simulink model "untitled1"  (Simulink 6.0)
settings: Solver=ode45  StartTime=0.0  StopTime=2  RelTol=1e-3
libraries: powerlib x5, powerlib_extras x3, simulink x1
settings Model: Creator=Daniel  LastModifiedBy=GXP
settings OptimizationCC: InlineInvariantSignals=off  InitFltsAndDblsToZero=off
settings DebuggingCC: SignalResolutionControl=UseLocalSettings
settings GRTTargetCC: TargetFcnLib=ansi_tfl_table_tmw.mat

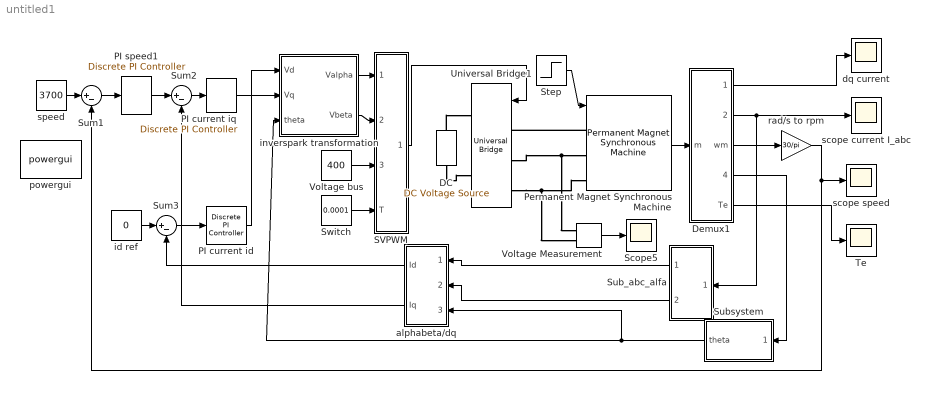
== system untitled1 ==
  " rad/s to rpm" : Gain  Gain=30/pi  ParameterDataType=fixdt(1, 16)  OutDataType=fixdt(1, 16)
  DC : powerlib/Electrical Sources/DC Voltage Source  Orientation=up  Amplitude=400  Measurements=Voltage
  Demux1 : Subsystem
  PI current id : powerlib_extras/Discrete  Control Blocks/Discrete PI Controller  Kp=100  Ki=7000  Par_Limits=[1000 -1000]  Init=0  Ts=50e-6
  PI current iq : powerlib_extras/Discrete  Control Blocks/Discrete PI Controller  Kp=100  Ki=7000  Par_Limits=[1000 -1000]  Init=0  Ts=50e-6
  PI speed1 : powerlib_extras/Discrete  Control Blocks/Discrete PI Controller  Kp=0.09  Ki=2.7  Par_Limits=[1500 -150]  Init=0  Ts=50e-6
  Permanent Magnet Synchronous Machine : powerlib/Machines/Permanent Magnet Synchronous Machine  PresetModel=No  ShowDetailedParameters=on  Resistance=1.08  Inductances=[8.5e-3, 8.5e-3]  Flux=0.1801  Mechanical=[0.00138 0.003 3]
  SVPWM : Subsystem
  Scope5 : Scope
      settings: TickLabels=on  TimeRange=2  YMin=-450  YMax=450  SaveName=ScopeData2  SampleInput=on
  Step : Step  Time=0.8  After=0  SampleTime=0
  Sub_abc_alfa : Subsystem  Orientation=left
  Subsystem : Subsystem  Orientation=left
  Sum1 : Sum  Inputs=|+-  OutDataType=fixdt(1, 16)
  Sum2 : Sum  Inputs=|+-  OutDataType=fixdt(1, 16)
  Sum3 : Sum  Inputs=|+-  OutDataType=fixdt(1, 16)
  Switch : Constant  Value=0.0001  VectorParams1D=off
  Te : Scope
      settings: TickLabels=on  TimeRange=1  YMin=1.9  YMax=2.5  SaveName=te3  SampleInput=on
  Universal Bridge1 : powerlib/Power Electronics/Universal Bridge  Orientation=left  Arms=3  SnubberResistance=1e5  SnubberCapacitance=inf  Device=IGBT / Diodes  Ron=1e-3  Lon=0  ForwardVoltages="[  0  0  ]"  ForwardVoltage=0  GTOparameters=[ 10e-6 , 20e-6 ]  IGBTparameters=[ 1e-6 , 2e-6 ]  Measurements=None
  Voltage Measurement : powerlib/Measurements/Voltage Measurement  PhasorSimulation=off  OutputType=Complex  PSBequivalent=0
  Voltage bus : Constant  Value=400  OutDataType=fixdt(1, 16)
  alphabeta/dq : Subsystem  Orientation=left
  dq current : Scope
      settings: TimeRange=2  YMin=-0.25  YMax=3.25  SaveName=ScopeData4  SampleInput=on
  id ref : Constant  Value=0
  inverspark transformation : Subsystem
  powergui : powerlib/powergui  Priority=2  Frange=[0:2:500]  Ylog=off  Xlog=on  save=off  variable=ZData  ZoomFFT=on  StartTime=0.0  cycles=1  DisplayStyle=1  fundamental=60  FreqAxis=off  MaxFrequency=1000  frequencyindice=0  frequencyindicesteady=1  RmsSteady=1  display=off  Ts=0  methode=off  frequency=60  echomessages=off
  scope current I_abc : Scope
      settings: TickLabels=on  TimeRange=2  YMin=-1.12119  YMax=0.92681  SaveName=ScopeData5  SampleInput=on
  scope speed : Scope
      settings: TimeRange=2  YMin=3740  YMax=3900  SaveName=ScopeData6  SampleInput=on
  speed : Constant  Value=3700
  wires:
  Sum1/1 -> PI speed1/1
  Sum2/1 -> PI current iq/1
  Sum3/1 -> PI current id/1
  Step/1 -> Permanent Magnet Synchronous Machine/1
  Voltage bus/1 -> SVPWM/3(Vdc)
  Switch/1 -> SVPWM/4(T)
  PI current id/1 -> inverspark transformation/1(Vd)
  PI current iq/1 -> inverspark transformation/2(Vq)
  Permanent Magnet Synchronous Machine/1 -> Demux1/1(m)
  Demux1/1(Is_dq) -> dq current/1
  Sub_abc_alfa/2(I_beeta) -> alphabeta/dq/2(I_beta)
  Demux1/4(theta) -> Subsystem/1(thetam)
  Demux1/2(Is_abc) -> Sub_abc_alfa/1(Is_abc), scope current I_abc/1
  Demux1/5(Te) -> Te/1
  Voltage Measurement/1 -> Scope5/1
  speed/1 -> Sum1/1
  Demux1/3(wm) -> " rad/s to rpm"/1
  " rad/s to rpm"/1 -> scope speed/1, Sum1/2
  inverspark transformation/1(Valpha) -> SVPWM/1(Valpha)
  inverspark transformation/2(Vbeta) -> SVPWM/2(Vbate)
  Subsystem/1(theta) -> alphabeta/dq/3(theta), inverspark transformation/3(theta)
  PI speed1/1 -> Sum2/1
  Sub_abc_alfa/1(I_alfa) -> alphabeta/dq/1(I_alpha)
  alphabeta/dq/1(Id) -> Sum3/2
  alphabeta/dq/2(Iq) -> Sum2/2
  SVPWM/1(Pules) -> Universal Bridge1/1
  id ref/1 -> Sum3/1
  connections:
  DC/RConn1 -- Universal Bridge1/RConn1
  DC/LConn1 -- Universal Bridge1/RConn2
  Universal Bridge1/LConn2 -- Permanent Magnet Synchronous Machine/LConn2 -- Voltage Measurement/LConn1
  Universal Bridge1/LConn3 -- Permanent Magnet Synchronous Machine/LConn3 -- Voltage Measurement/LConn2
  Permanent Magnet Synchronous Machine/LConn1 -- Universal Bridge1/LConn1

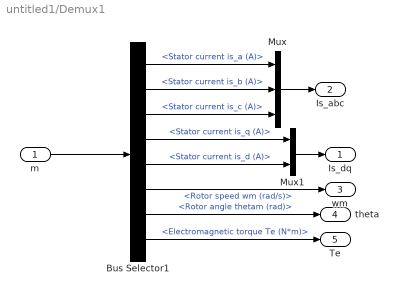
== system untitled1/Demux1 ==
  m : Inport  Port=1  LatchInput=off
  Bus Selector1 : BusSelector  DialogController=Simulink.DDGSource_Bus  OutputSignals=Stator current is_a (A),Stator current is_b (A),Stator current is_c (A),Stator current is_q (A),Stator current is_d (A),Rotor speed wm (rad/s),Rotor angle thetam (rad),Electromagnetic torque Te (N*m)
  Mux : Mux  Inputs=3
  Mux1 : Mux  Inputs=2
  Is_dq : Outport
  Is_abc : Outport  Port=2
  wm : Outport  Port=3
  theta : Outport  Port=4
  Te : Outport  Port=5
  wires:
  m/1 -> Bus Selector1/1
  Bus Selector1/1 -> Mux/1  "<Stator current is_a (A)>"
  Bus Selector1/2 -> Mux/2  "<Stator current is_b (A)>"
  Bus Selector1/3 -> Mux/3  "<Stator current is_c (A)>"
  Bus Selector1/6 -> wm/1  "<Rotor speed wm (rad/s)>"
  Bus Selector1/7 -> theta/1  "<Rotor angle thetam (rad)>"
  Bus Selector1/8 -> Te/1  "<Electromagnetic torque Te (N*m)>"
  Mux/1 -> Is_abc/1
  Bus Selector1/5 -> Mux1/2  "<Stator current is_d (A)>"
  Bus Selector1/4 -> Mux1/1  "<Stator current is_q (A)>"
  Mux1/1 -> Is_dq/1

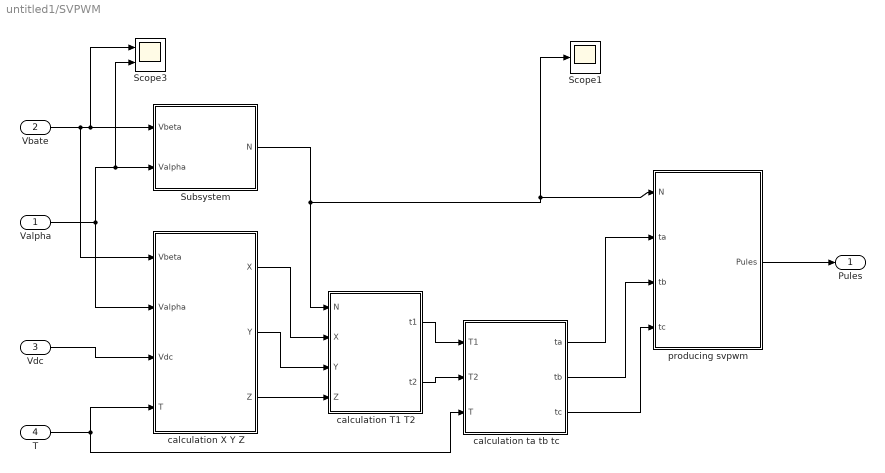
== system untitled1/SVPWM ==
  Valpha : Inport  Port=1  OutDataType=fixdt(1, 16)  LatchInput=off
  Vbate : Inport  Port=2  OutDataType=fixdt(1, 16)  LatchInput=off
  Vdc : Inport  Port=3  OutDataType=fixdt(1, 16)  LatchInput=off
  T : Inport  Port=4  OutDataType=fixdt(1, 16)  LatchInput=off
  Scope1 : Scope
      settings: YMin=1  YMax=6
  Scope3 : Scope  NumInputPorts=2
      settings: TimeRange=0.1  YMin=-250~-275  YMax=250~275
  Subsystem : Subsystem
  calculation T1 T2 : Subsystem
  calculation X Y Z : Subsystem
  calculation ta tb tc : Subsystem
  producing svpwm : Subsystem
  Pules : Outport  OutDataType=fixdt(1, 16)
  wires:
  Vbate/1 -> calculation X Y Z/1(Vbeta), Subsystem/1(Vbeta), Scope3/1
  Valpha/1 -> calculation X Y Z/2(Valpha), Subsystem/2(Valpha), Scope3/2
  Vdc/1 -> calculation X Y Z/3(Vdc)
  T/1 -> calculation X Y Z/4(T), calculation ta tb tc/3(T)
  calculation X Y Z/1(X) -> calculation T1 T2/2(X)
  calculation X Y Z/2(Y) -> calculation T1 T2/3(Y)
  calculation X Y Z/3(Z) -> calculation T1 T2/4(Z)
  Subsystem/1(N) -> calculation T1 T2/1(N), Scope1/1, producing svpwm/1(N)
  calculation ta tb tc/1(ta) -> producing svpwm/2(ta)
  calculation ta tb tc/2(tb) -> producing svpwm/3(tb)
  calculation ta tb tc/3(tc) -> producing svpwm/4(tc)
  producing svpwm/1(Pules) -> Pules/1
  calculation T1 T2/2(t2) -> calculation ta tb tc/2(T2)
  calculation T1 T2/1(t1) -> calculation ta tb tc/1(T1)

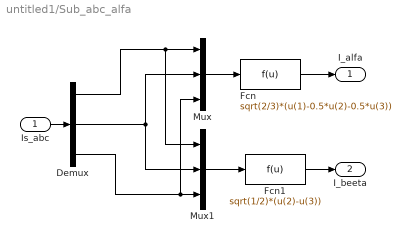
== system untitled1/Sub_abc_alfa ==
  Is_abc : Inport  Port=1  LatchInput=off
  Demux : Demux  Outputs=3
  Fcn : Fcn  Expr=sqrt(2/3)*(u(1)-0.5*u(2)-0.5*u(3))
  Fcn1 : Fcn  Expr=sqrt(1/2)*(u(2)-u(3))
  Mux : Mux  Inputs=3
  Mux1 : Mux  Inputs=3
  I_alfa : Outport
  I_beeta : Outport  Port=2
  wires:
  Is_abc/1 -> Demux/1
  Demux/1 -> Mux/1, Mux1/1
  Mux/1 -> Fcn/1
  Mux1/1 -> Fcn1/1
  Demux/3 -> Mux/3, Mux1/3
  Demux/2 -> Mux/2, Mux1/2
  Fcn/1 -> I_alfa/1
  Fcn1/1 -> I_beeta/1

== system untitled1/Subsystem ==
  thetam : Inport  Port=1  OutDataType=fixdt(1, 16)  LatchInput=off
  Add1 : Sum  Inputs=+-  OutDataType=fixdt(1,16,0)  OutScaling=[]
  Constant4 : Constant  Value=0.5*pi  OutDataType=fixdt(1,16,0)  OutScaling=[]
  Gain1 : Gain  Gain=3  ParameterDataType=fixdt(1,16,0)  ParameterScaling=[]  OutDataType=fixdt(1,16,0)  OutScaling=[]
  theta : Outport  OutDataType=fixdt(1, 16)
  wires:
  Gain1/1 -> Add1/1
  Constant4/1 -> Add1/2
  Add1/1 -> theta/1
  thetam/1 -> Gain1/1

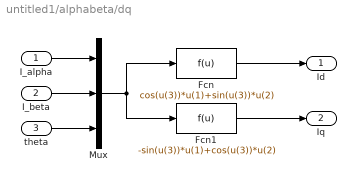
== system untitled1/alphabeta/dq ==
  I_alpha : Inport  Port=1  LatchInput=off
  I_beta : Inport  Port=2  LatchInput=off
  theta : Inport  Port=3  LatchInput=off
  Fcn : Fcn  Expr=cos(u(3))*u(1)+sin(u(3))*u(2)
  Fcn1 : Fcn  Expr=-sin(u(3))*u(1)+cos(u(3))*u(2)
  Mux : Mux  Inputs=3
  Id : Outport
  Iq : Outport  Port=2
  wires:
  I_alpha/1 -> Mux/1
  I_beta/1 -> Mux/2
  theta/1 -> Mux/3
  Mux/1 -> Fcn/1, Fcn1/1
  Fcn/1 -> Id/1
  Fcn1/1 -> Iq/1

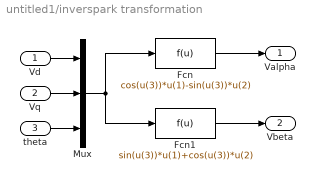
== system untitled1/inverspark transformation ==
  Vd : Inport  Port=1  LatchInput=off
  Vq : Inport  Port=2  LatchInput=off
  theta : Inport  Port=3  LatchInput=off
  Fcn : Fcn  Expr=cos(u(3))*u(1)-sin(u(3))*u(2)
  Fcn1 : Fcn  Expr=sin(u(3))*u(1)+cos(u(3))*u(2)
  Mux : Mux  Inputs=3
  Valpha : Outport
  Vbeta : Outport  Port=2
  wires:
  Vd/1 -> Mux/1
  Vq/1 -> Mux/2
  theta/1 -> Mux/3
  Mux/1 -> Fcn/1, Fcn1/1
  Fcn/1 -> Valpha/1
  Fcn1/1 -> Vbeta/1

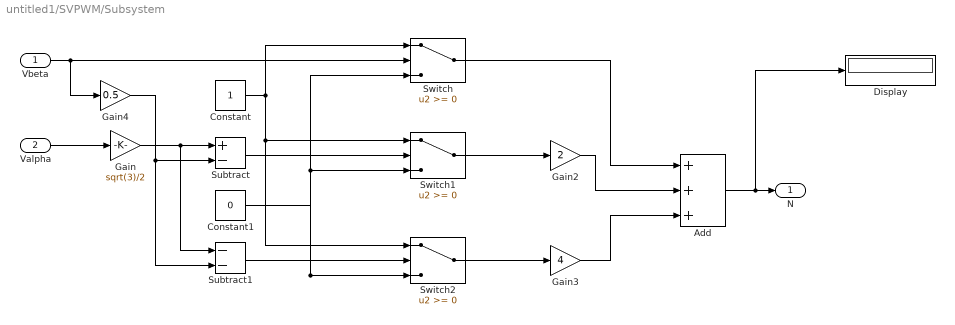
== system untitled1/SVPWM/Subsystem ==
  Vbeta : Inport  Port=1  OutDataType=fixdt(1, 16)  LatchInput=off
  Valpha : Inport  Port=2  OutDataType=fixdt(1, 16)  LatchInput=off
  Add : Sum  Inputs=+++  OutDataType=fixdt(1, 16)  OutScaling=2^-10
  Constant : Constant  OutDataType=fixdt(1, 16)
  Constant1 : Constant  Value=0  OutDataType=fixdt(1, 16)
  Display : Display
  Gain : Gain  Gain=sqrt(3)/2
  Gain2 : Gain  Gain=2  ParameterDataType=fixdt(1, 16)  OutDataType=fixdt(1, 16)
  Gain3 : Gain  Gain=4  ParameterDataType=fixdt(1, 16)  OutDataType=fixdt(1, 16)
  Gain4 : Gain  Gain=0.5
  Subtract : Sum  Inputs=+-  OutDataType=fixdt(1, 16)  OutScaling=2^-10
  Subtract1 : Sum  Inputs=--  OutDataType=fixdt(1, 16)  OutScaling=2^-10
  Switch : Switch
  Switch1 : Switch
  Switch2 : Switch
  N : Outport  OutDataType=fixdt(1, 16)
  wires:
  Valpha/1 -> Gain/1
  Vbeta/1 -> Switch/2, Gain4/1
  Subtract/1 -> Switch1/2
  Subtract1/1 -> Switch2/2
  Constant/1 -> Switch/1, Switch1/1, Switch2/1
  Constant1/1 -> Switch/3, Switch1/3, Switch2/3
  Switch1/1 -> Gain2/1
  Switch2/1 -> Gain3/1
  Switch/1 -> Add/1
  Gain2/1 -> Add/2
  Gain3/1 -> Add/3
  Add/1 -> N/1, Display/1
  Gain/1 -> Subtract/1, Subtract1/1
  Gain4/1 -> Subtract/2, Subtract1/2

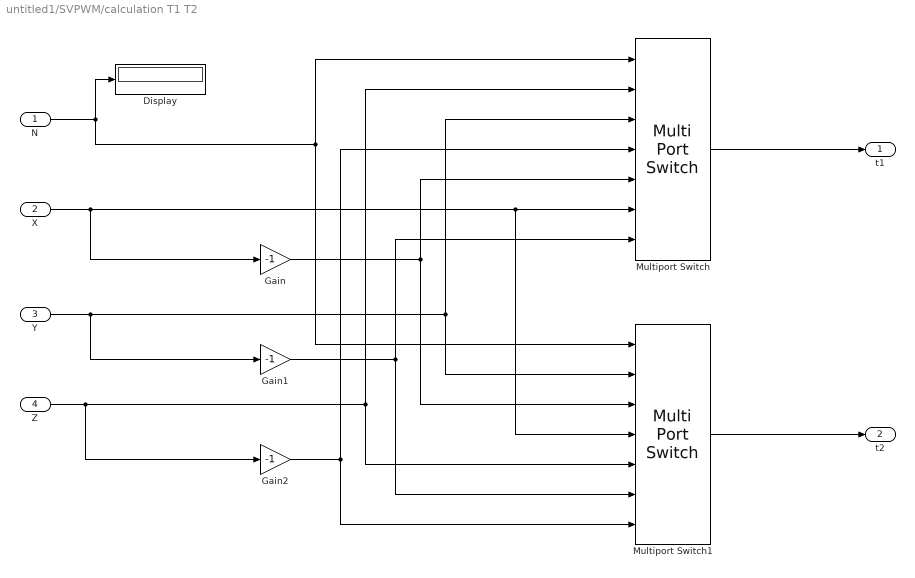
== system untitled1/SVPWM/calculation T1 T2 ==
  N : Inport  Port=1  OutDataType=fixdt(1, 16)  LatchInput=off
  X : Inport  Port=2  OutDataType=fixdt(1, 16)  LatchInput=off
  Y : Inport  Port=3  OutDataType=fixdt(1, 16)  LatchInput=off
  Z : Inport  Port=4  OutDataType=fixdt(1, 16)  LatchInput=off
  Display : Display
  Gain : Gain  Gain=-1  ParameterDataType=fixdt(1, 16)  OutDataType=fixdt(1, 16)
  Gain1 : Gain  Gain=-1  ParameterDataType=fixdt(1, 16)  OutDataType=fixdt(1, 16)
  Gain2 : Gain  Gain=-1  ParameterDataType=fixdt(1, 16)  OutDataType=fixdt(1, 16)
  Multiport Switch : MultiPortSwitch  Inputs=6
  Multiport Switch1 : MultiPortSwitch  Inputs=6
  t1 : Outport
  t2 : Outport  Port=2
  wires:
  N/1 -> Multiport Switch/1, Multiport Switch1/1, Display/1
  Z/1 -> Multiport Switch/2, Multiport Switch1/5, Gain2/1
  Y/1 -> Gain1/1, Multiport Switch1/2, Multiport Switch/3
  Gain2/1 -> Multiport Switch/4, Multiport Switch1/7
  Gain/1 -> Multiport Switch/5, Multiport Switch1/3
  X/1 -> Multiport Switch/6, Multiport Switch1/4, Gain/1
  Gain1/1 -> Multiport Switch/7, Multiport Switch1/6
  Multiport Switch1/1 -> t2/1
  Multiport Switch/1 -> t1/1

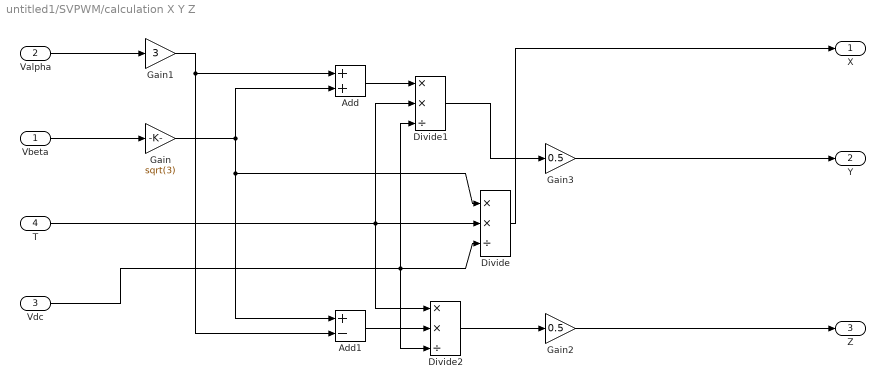
== system untitled1/SVPWM/calculation X Y Z ==
  Vbeta : Inport  Port=1  OutDataType=fixdt(1, 16)  LatchInput=off
  Valpha : Inport  Port=2  OutDataType=fixdt(1, 16)  LatchInput=off
  Vdc : Inport  Port=3  OutDataType=fixdt(1, 16)  LatchInput=off
  T : Inport  Port=4  OutDataType=fixdt(1, 16)  LatchInput=off
  Add : Sum  OutScaling=2^-10
  Add1 : Sum  Inputs=+-  OutScaling=2^-10
  Divide : Product  Inputs=**/  OutScaling=2^-10
  Divide1 : Product  Inputs=**/  OutScaling=2^-10
  Divide2 : Product  Inputs=**/  OutScaling=2^-10
  Gain : Gain  Gain=sqrt(3)
  Gain1 : Gain  Gain=3
  Gain2 : Gain  Gain=0.5
  Gain3 : Gain  Gain=0.5
  X : Outport  OutDataType=fixdt(1, 16)
  Y : Outport  Port=2  OutDataType=fixdt(1, 16)
  Z : Outport  Port=3  OutDataType=fixdt(1, 16)
  wires:
  Vbeta/1 -> Gain/1
  Gain/1 -> Add/2, Divide/1, Add1/1
  T/1 -> Divide/2, Divide1/2, Divide2/1
  Vdc/1 -> Divide/3, Divide1/3, Divide2/3
  Valpha/1 -> Gain1/1
  Gain1/1 -> Add/1, Add1/2
  Add/1 -> Divide1/1
  Add1/1 -> Divide2/2
  Divide2/1 -> Gain2/1
  Gain2/1 -> Z/1
  Divide/1 -> X/1
  Divide1/1 -> Gain3/1
  Gain3/1 -> Y/1

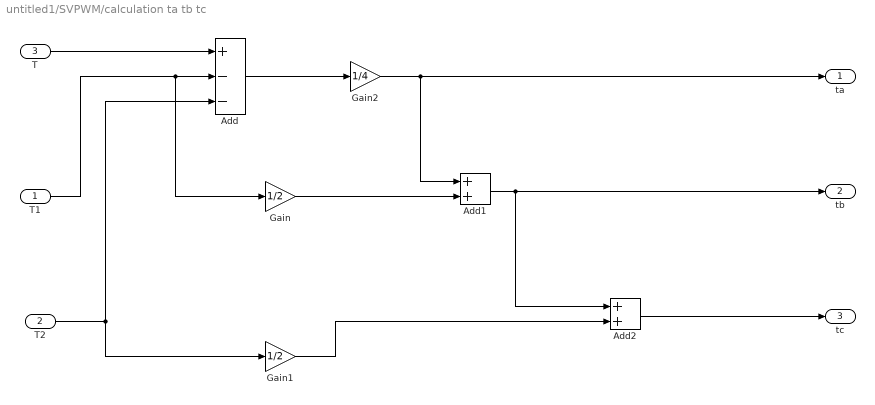
== system untitled1/SVPWM/calculation ta tb tc ==
  T1 : Inport  Port=1  OutDataType=fixdt(1, 16)  LatchInput=off
  T2 : Inport  Port=2  OutDataType=fixdt(1, 16)  LatchInput=off
  T : Inport  Port=3  OutDataType=fixdt(1, 16)  LatchInput=off
  Add : Sum  Inputs=+--  OutDataType=fixdt(1, 16)  OutScaling=2^-10
  Add1 : Sum  OutDataType=fixdt(1, 16)  OutScaling=2^-10
  Add2 : Sum  OutDataType=fixdt(1, 16)  OutScaling=2^-10
  Gain : Gain  Gain=1/2  ParameterDataType=fixdt(1, 16)  OutDataType=fixdt(1, 16)
  Gain1 : Gain  Gain=1/2  ParameterDataType=fixdt(1, 16)  OutDataType=fixdt(1, 16)
  Gain2 : Gain  Gain=1/4  ParameterDataType=fixdt(1, 16)  OutDataType=fixdt(1, 16)
  ta : Outport  OutDataType=fixdt(1, 16)
  tb : Outport  Port=2  OutDataType=fixdt(1, 16)
  tc : Outport  Port=3  OutDataType=fixdt(1, 16)
  wires:
  T/1 -> Add/1
  T1/1 -> Add/2, Gain/1
  T2/1 -> Add/3, Gain1/1
  Add/1 -> Gain2/1
  Gain/1 -> Add1/2
  Gain2/1 -> ta/1, Add1/1
  Add1/1 -> tb/1, Add2/1
  Add2/1 -> tc/1
  Gain1/1 -> Add2/2

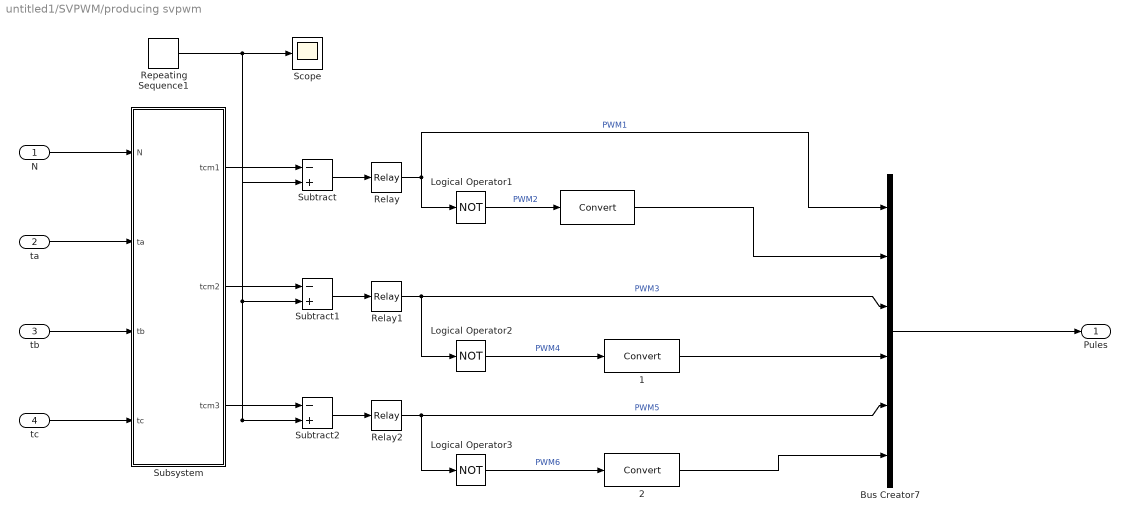
== system untitled1/SVPWM/producing svpwm ==
  N : Inport  Port=1  OutDataType=fixdt(1, 16)  LatchInput=off
  ta : Inport  Port=2  OutDataType=fixdt(1, 16)  LatchInput=off
  tb : Inport  Port=3  OutDataType=fixdt(1, 16)  LatchInput=off
  tc : Inport  Port=4  OutDataType=fixdt(1, 16)  LatchInput=off
  "  " : DataTypeConversion  OutDataTypeMode=double
  "  1" : DataTypeConversion  OutDataTypeMode=double
  "  2" : DataTypeConversion  OutDataTypeMode=double
  Bus Creator7 : BusCreator  DialogController=Simulink.DDGSource_Bus  Inputs=6
  Logical Operator1 : Logic  Operator=NOT  AllPortsSameDT=off  LogicDataType=float('double')
  Logical Operator2 : Logic  Operator=NOT  AllPortsSameDT=off  LogicDataType=float('double')
  Logical Operator3 : Logic  Operator=NOT  AllPortsSameDT=off  LogicDataType=float('double')
  Relay : Relay  OutDataType=fixdt(1, 16)
  Relay1 : Relay  OutDataType=fixdt(1, 16)
  Relay2 : Relay  OutDataType=fixdt(1, 16)
  Repeating Sequence1 : simulink/Sources/Repeating Sequence  rep_seq_t=[0 0.0001/2 0.0001]  rep_seq_y=[0 0.0001/2 0]
  Scope : Scope
      settings: TimeRange=0.4  YMin=2e-005  YMax=8e-005  SaveName=ScopeData3
  Subsystem : Subsystem
  Subtract : Sum  Inputs=-+  OutDataType=fixdt(1, 16)  OutScaling=2^-10
  Subtract1 : Sum  Inputs=-+  OutDataType=fixdt(1, 16)  OutScaling=2^-10
  Subtract2 : Sum  Inputs=-+  OutDataType=fixdt(1, 16)  OutScaling=2^-10
  Pules : Outport  OutDataType=fixdt(1, 16)
  wires:
  N/1 -> Subsystem/1(N)
  ta/1 -> Subsystem/2(ta)
  tb/1 -> Subsystem/3(tb)
  tc/1 -> Subsystem/4(tc)
  Subsystem/1(tcm1) -> Subtract/1
  Subsystem/2(tcm2) -> Subtract1/1
  Subsystem/3(tcm3) -> Subtract2/1
  Repeating Sequence1/1 -> Subtract/2, Subtract1/2, Subtract2/2, Scope/1
  Subtract/1 -> Relay/1
  Subtract1/1 -> Relay1/1
  Subtract2/1 -> Relay2/1
  Relay/1 -> Logical Operator1/1, Bus Creator7/1  "PWM1"
  Relay1/1 -> Logical Operator2/1, Bus Creator7/3  "PWM3"
  Relay2/1 -> Logical Operator3/1, Bus Creator7/5  "PWM5"
  Bus Creator7/1 -> Pules/1
  "  "/1 -> Bus Creator7/2
  Logical Operator1/1 -> "  "/1  "PWM2"
  Logical Operator2/1 -> "  1"/1  "PWM4"
  "  1"/1 -> Bus Creator7/4
  Logical Operator3/1 -> "  2"/1  "PWM6"
  "  2"/1 -> Bus Creator7/6

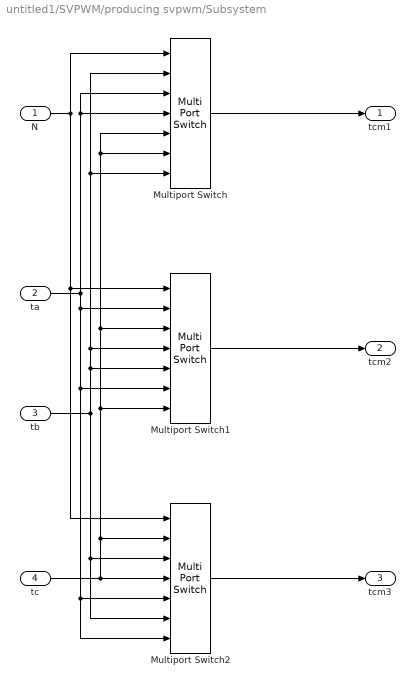
== system untitled1/SVPWM/producing svpwm/Subsystem ==
  N : Inport  Port=1  OutDataType=fixdt(1, 16)  LatchInput=off
  ta : Inport  Port=2  OutDataType=fixdt(1, 16)  LatchInput=off
  tb : Inport  Port=3  OutDataType=fixdt(1, 16)  LatchInput=off
  tc : Inport  Port=4  OutDataType=fixdt(1, 16)  LatchInput=off
  Multiport Switch : MultiPortSwitch  Inputs=6
  Multiport Switch1 : MultiPortSwitch  Inputs=6
  Multiport Switch2 : MultiPortSwitch  Inputs=6
  tcm1 : Outport  OutDataType=fixdt(1, 16)
  tcm2 : Outport  Port=2  OutDataType=fixdt(1, 16)
  tcm3 : Outport  Port=3  OutDataType=fixdt(1, 16)
  wires:
  N/1 -> Multiport Switch/1, Multiport Switch1/1, Multiport Switch2/1
  ta/1 -> Multiport Switch/3, Multiport Switch/4, Multiport Switch1/2, Multiport Switch1/6, Multiport Switch2/5, Multiport Switch2/7
  tb/1 -> Multiport Switch/2, Multiport Switch/7, Multiport Switch1/4, Multiport Switch1/5, Multiport Switch2/3, Multiport Switch2/6
  tc/1 -> Multiport Switch2/4, Multiport Switch2/2, Multiport Switch/5, Multiport Switch/6, Multiport Switch1/3, Multiport Switch1/7
  Multiport Switch/1 -> tcm1/1
  Multiport Switch1/1 -> tcm2/1
  Multiport Switch2/1 -> tcm3/1
